simulink library "linearLeastSqrs_ul"  (R2020a)
settings: Solver=VariableStepAuto  StartTime=0.0  StopTime=10.0  RelTol=1e-3
settings Model: Creator=mcobb  LastModifiedBy=mitch
settings DataIOCC: ReturnWorkspaceOutputs=off
settings DebuggingCC: ArithmeticOperatorsInVariantConditions=warning
settings SFSimCC: CustomCodeUndefinedFunction=UseInterfaceOnly

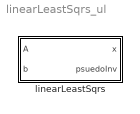
== system linearLeastSqrs_ul ==
  linearLeastSqrs : Subsystem

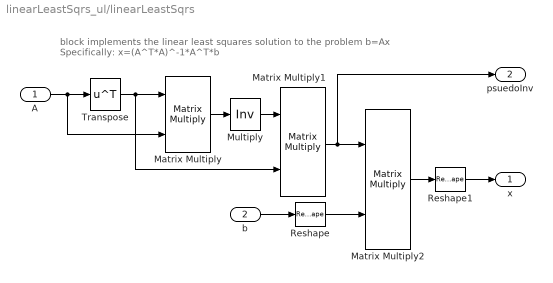
== system linearLeastSqrs_ul/linearLeastSqrs ==
  note: block implements the linear least squares solution to the problem b=Ax
      | Specifically: x=(A^T*A)^-1*A^T*b
  A : Inport
  b : Inport  Port=2
  Matrix Multiply : Product  Multiplication=Matrix(*)
  Matrix Multiply1 : Product  Multiplication=Matrix(*)
  Matrix Multiply2 : Product  Multiplication=Matrix(*)
  Multiply : Product  Inputs=/  Multiplication=Matrix(*)
  Reshape : Reshape  OutputDimensionality=Column vector (2-D)
  Reshape1 : Reshape  OutputDimensionality=Column vector (2-D)
  Transpose : Math  Operator=transpose  SignedPower=on  SaturateOnIntegerOverflow=on
  x : Outport  VectorParamsAs1DForOutWhenUnconnected=off
  psuedoInv : Outport  Port=2  VectorParamsAs1DForOutWhenUnconnected=off
  wires:
  A/1 -> Matrix Multiply/2, Transpose/1
  Matrix Multiply/1 -> Multiply/1
  Multiply/1 -> Matrix Multiply1/1
  Transpose/1 -> Matrix Multiply1/2, Matrix Multiply/1
  b/1 -> Reshape/1
  Matrix Multiply1/1 -> Matrix Multiply2/1, psuedoInv/1
  Reshape/1 -> Matrix Multiply2/2
  Reshape1/1 -> x/1
  Matrix Multiply2/1 -> Reshape1/1
